simulink model "Van_der_Pol"  (R2020a)
settings: Solver=VariableStepAuto  StartTime=0.0  StopTime=20  RelTol=1e-3
settings Model: Creator=BEAR  LastModifiedBy=bzhan
settings DataIOCC: ReturnWorkspaceOutputs=off
settings DebuggingCC: ArithmeticOperatorsInVariantConditions=warning
settings SFSimCC: SimUseLocalCustomCode=off  CustomCodeUndefinedFunction=UseInterfaceOnly
settings RTWCC: RTWUseLocalCustomCode=off

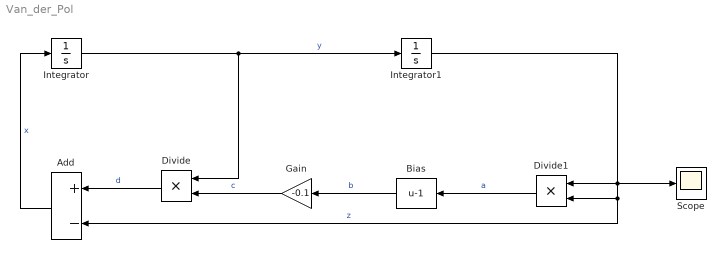
== system Van_der_Pol ==
  Add : Sum  Inputs=+-
  Bias : Bias  Bias=-1
  Divide : Product  Inputs=**
  Divide1 : Product  Inputs=**  SampleTime=6
  Gain : Gain  Gain=-0.1  SampleTime=4
  Integrator : Integrator  InitialCondition=1
  Integrator1 : Integrator  InitialCondition=1
  Scope : Scope
  wires:
  Add/1 -> Integrator/1  "x"
  Divide/1 -> Add/1  "d"
  Integrator/1 -> Divide/1, Integrator1/1  "y"
  Gain/1 -> Divide/2  "c"
  Bias/1 -> Gain/1  "b"
  Divide1/1 -> Bias/1  "a"
  Integrator1/1 -> Scope/1, Divide1/1, Divide1/2, Add/2  "z"
